simulink model "experiment_1_lab_05_e"  (Simulink 7.1)
settings: Solver=ode45  StartTime=0.0  StopTime=10.0  RelTol=1e-3
InitFcn:
  | R1=2;
  | R2=4;
  | L1=0.5;
  | L2=1;
  | C=3/8;
  | A=[-R1/L1,0,-1/L1;0,-R2/L2,1/L2;1/C,-1/C,0];
  | B= [1/L1;0;0];
  | C=[0,R2,0;1,0,0;0,1,0;0,0,1;1,-1,0;-R1,0,-1];
  | D=[0;0;0;0;0;1];
  | 
  | [Q2 L] = eig(A);
  | 
  | Q3=[real(Q2(:,1)),imag(Q2(:,1)),Q2(:,3)];
  | AB=Q3*A*inv(Q3);
  | BB=Q3*B;
  | CB=C*inv(Q3);
  | DB=[0;0;0;0;0;1];
settings Model: Creator=ALUNO  LastModifiedBy=ALUNO

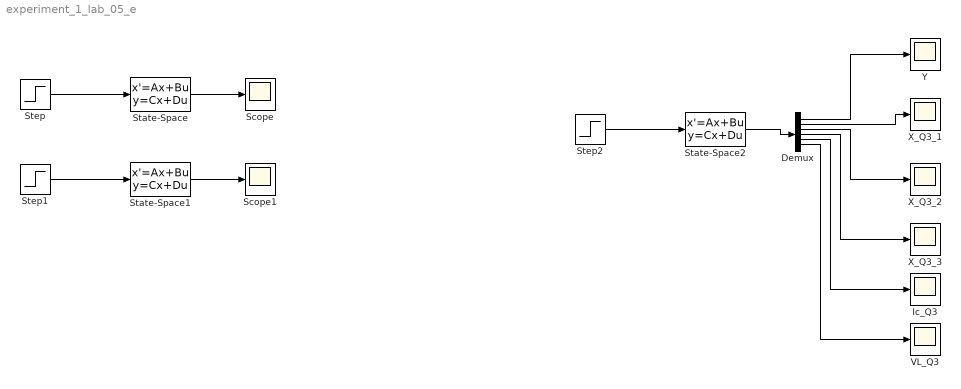
== system experiment_1_lab_05_e ==
  Demux : Demux  Outputs=6
  Ic_Q3 : Scope
      settings: SaveName=ScopeData2
  Scope : Scope
  Scope1 : Scope
  State-Space : StateSpace  A=AB  B=BB  C=CB  D=DB
  State-Space1 : StateSpace  A=A  B=B  C=C  D=D
  State-Space2 : StateSpace  A=AB  B=BB  C=CB  D=DB
  Step : Step  Time=0  SampleTime=0
  Step1 : Step  Time=0  SampleTime=0
  Step2 : Step  Time=0  SampleTime=0
  VL_Q3 : Scope
      settings: SaveName=ScopeData7
  X_Q3_1 : Scope
      settings: SaveName=ScopeData5
  X_Q3_2 : Scope
      settings: SaveName=ScopeData6
  X_Q3_3 : Scope
      settings: SaveName=ScopeData3
  Y : Scope
      settings: SaveName=ScopeData4
  wires:
  Step/1 -> State-Space/1
  State-Space/1 -> Scope/1
  Step1/1 -> State-Space1/1
  State-Space1/1 -> Scope1/1
  Step2/1 -> State-Space2/1
  State-Space2/1 -> Demux/1
  Demux/1 -> Y/1
  Demux/2 -> X_Q3_1/1
  Demux/3 -> X_Q3_2/1
  Demux/4 -> X_Q3_3/1
  Demux/5 -> Ic_Q3/1
  Demux/6 -> VL_Q3/1
